simulink model "untitled1"  (R2025b)
settings: Solver=VariableStepAuto  StartTime=0.0  StopTime=10.0  RelTol=1e-3
libraries: simulink x1
settings Model: Creator=marie  LastModifiedBy=marie

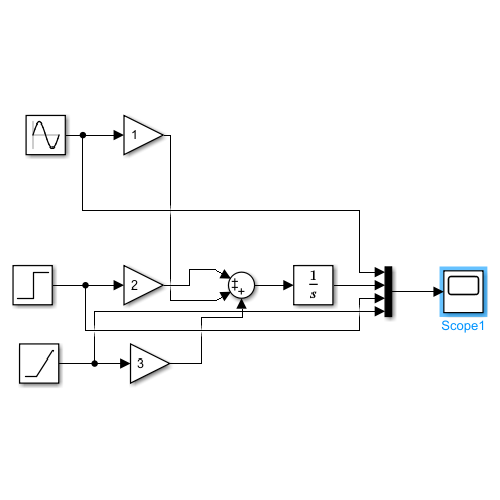
[thumbnail: Simulink's stored preview of the top-level diagram]
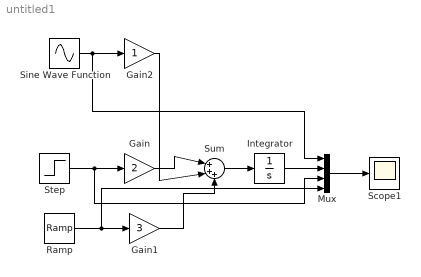
== system untitled1 ==
  Gain : Gain  Gain=2
  Gain1 : Gain  Gain=3
  Gain2 : Gain
  Integrator : Integrator
  Mux : Mux
  Ramp : simulink/Sources/Ramp  slope=1  start=0  InitialOutput=0
  Scope1 : Scope
      settings: ActiveDisplayYMinimum=0.27080645705490003  ActiveDisplayYMaximum=16.789802095231842
  Sine Wave Function : Sin  Amplitude=10  Frequency=7  Phase=3  Samples=3  SampleTime=0  Offset=5
  Step : Step  Time=0  After=4  SampleTime=0
  Sum : Sum  Inputs=|+++
  wires:
  Sum/1 -> Integrator/1
  Step/1 -> Mux/3, Gain/1
  Ramp/1 -> Mux/4, Gain1/1
  Gain/1 -> Sum/1
  Gain1/1 -> Sum/3
  Sine Wave Function/1 -> Mux/1, Gain2/1
  Gain2/1 -> Sum/2
  Integrator/1 -> Mux/2
  Mux/1 -> Scope1/1
